simulink model "M_QAM"  (Simulink 8.1)
settings: Solver=ode45  StartTime=0.0  StopTime=20.0  RelTol=1e-3
undefined symbols (not defined in the file or in its folder): get
libraries: commdigbbndam3 x2, commviewers2 x2, commchan3 x1, commsink2 x1, commrandsrc2 x1
settings Model: Creator=Ammar  LastModifiedBy=User

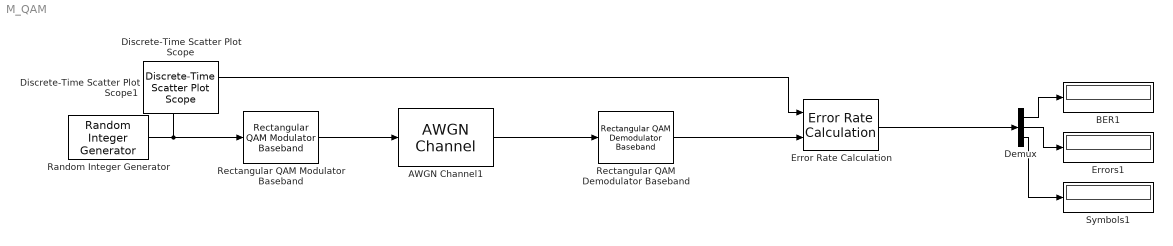
== system M_QAM ==
  AWGN Channel1 : commchan3/AWGN Channel  InputProcessing=Columns as channels (frame based)  seed=67  noiseMode="Signal to noise ratio  (Eb/No)"  EbNodB=1  EsNodB=3  SNRdB=3  bitsPerSym=4  Ps=1  Tsym=1/1000  variance=1
  BER1 : Display
  Demux : Demux  Outputs=3
  Error Rate Calculation : commsink2/Error Rate Calculation  N=0  st_delay=0  cp_mode=Entire frame  subframe=[]  PMode=Port  WsName=ErrorVec  RsMode2=off  stop=off  numErr=100  maxBits=1e6
  Errors1 : Display
  Random Integer Generator : commrandsrc2/Random Integer Generator  mul=16  seed=35  Ts=1/1000  frameBased=off  sampPerFrame=1  orient=off  outDataType=double
  Rectangular QAM Demodulator Baseband : commdigbbndam3/Rectangular QAM Demodulator Baseband  M=16  PowType=Min. distance between symbols  MinDist=2  AvgPow=1  PeakPow=1  Ph=0  Dec=Gray  Mapping=[0:15]  OutType=Integer  DecType=Hard decision  VarSource=Dialog  Variance=1  outDtype1=Inherit via internal rule  outDtype2=Inherit via internal rule  derotateFactorWordLen=16  denormFactorWordLen=16  prodOutWordLen=32  prodOutRoundingMode=Floor  prodOutOverflowMode=Wrap  sumWordLen=32
  Rectangular QAM Modulator Baseband : commdigbbndam3/Rectangular QAM Modulator Baseband  M=16  InType=Integer  Enc=Gray  Mapping=[0:15]  PowType=Min. distance between symbols  MinDist=2  AvgPow=1  PeakPow=1  Ph=0  outDtype=double  outWordLen=16  outUDDataType=sfix(16)  outFracLenMode=Best precision  outFracLen=15
  Symbols1 : Display
  Discrete-Time Scatter Plot Scope : commviewers2/Discrete-Time Scatter Plot Scope  Tag=ScatterPlot  IOType=viewer  sampPerSymb=1  offsetEye=0  numTraces=40  numNewFrames=10  LineMarkers=.  LineColors=b  fading=on  render=on  AxisGrid=on  xMin=-8.5  xMax=8.5  yMin=-8.5  yMax=8.5  inphaseLabel=In-phase Amplitude  quadratureLabel=Quadrature Amplitude  openScopeAtSimStart=on  FrameNumber=off  FigPos=get(0,'defaultfigureposition');  figTitle=Scatter Plot  numLinesMax=8  block_type_=scatter
  Discrete-Time Scatter Plot Scope1 : commviewers2/Discrete-Time Scatter Plot Scope  Tag=ScatterPlot  IOType=viewer  sampPerSymb=1  offsetEye=0  numTraces=40  numNewFrames=10  LineMarkers=.  LineColors=b  fading=on  render=on  AxisGrid=on  xMin=-8.5  xMax=8.5  yMin=-8.5  yMax=8.5  inphaseLabel=In-phase Amplitude  quadratureLabel=Quadrature Amplitude  openScopeAtSimStart=on  FrameNumber=off  FigPos=get(0,'defaultfigureposition');  figTitle=Scatter Plot  numLinesMax=8  block_type_=scatter
  wires:
  Random Integer Generator/1 -> Rectangular QAM Modulator Baseband/1, Error Rate Calculation/1
  Demux/1 -> BER1/1
  Demux/2 -> Errors1/1
  Demux/3 -> Symbols1/1
  Error Rate Calculation/1 -> Demux/1
  Rectangular QAM Modulator Baseband/1 -> AWGN Channel1/1
  AWGN Channel1/1 -> Rectangular QAM Demodulator Baseband/1
  Rectangular QAM Demodulator Baseband/1 -> Error Rate Calculation/2
